simulink model "mpc_utarget"  (Simulink 6.0)
settings: Solver=ode45  SolverMode=SingleTasking  StartTime=0.0  StopTime=5  RelTol=1e-3
values from neighbouring files (symbols this model uses):
  A = sys.a    [misosim.m]    (also in mpcutarget.m)
  B = sys.b    [misosim.m]    (also in mpcutarget.m)
  C = sys.c    [misosim.m]    (also in mpcutarget.m)
  D = sys.d    [misosim.m]    (also in mpcutarget.m)
  x0 = [0 0 0 0 0]'    [misosim.m]    (also in mpcmotormodel.m = zeros(4,1); mpcoutputconstr.m = [0 0]'; mpcpreview.m = [0 0 0]'; mpcutarget.m = [0 0 0 0]')
libraries: mpclib x1
settings Model: Creator=jowen  LastModifiedBy=jowen  ExtModeTrigMode=oneshot  ExtModeArmWhenConnect=off
settings DataIOCC: LimitDataPoints=off  SignalLoggingName=sigsOut
settings OptimizationCC: BooleanDataType=off
settings DebuggingCC: CheckExecutionContextPreStartOutputMsg=on  CheckExecutionContextRuntimeOutputMsg=on  SolverPrmCheckMsg=none  IntegerOverflowMsg=none
settings HardwareCC: TargetUnknown=on
settings SFSimCC: SFSimApplyToAllLibs=on  SFSimBuildMode=Incremental

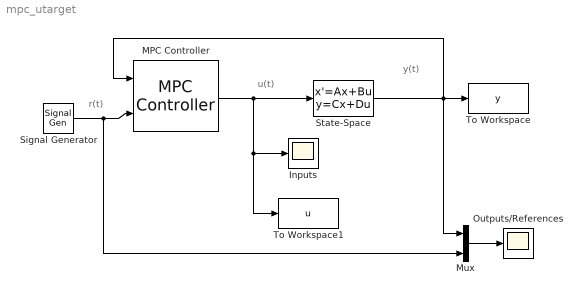
== system mpc_utarget ==
  note: u(t)
  note: y(t)
  note: r(t)
  Inputs : Scope
      settings: TimeRange=40  YMin=-4  YMax=3  DataFormat=Structure
  MPC Controller : mpclib/MPC Controller  mpcobj=mpcobj  n_mv=0  x0=[]  ref_from_ws=off  ref_signal_name=[]  ref_preview=on  md_from_ws=off  md_signal_name=[]  md_preview=on  from_project=off  md_inport=off  project_file=MPCtask.mat
  Mux : Mux  Inputs=2
  Outputs/References : Scope
      settings: TimeRange=40  YMin=-1.5  YMax=1.5  DataFormat=Structure
  Signal Generator : SignalGenerator  WaveForm=square  Frequency=.025
  State-Space : StateSpace  A=A  B=B  C=C  D=D  X0=x0
  To Workspace : ToWorkspace  VariableName=y  SampleTime=-1  SaveFormat=Array
      settings: MaxDataPoints=Inf
  To Workspace1 : ToWorkspace  VariableName=u  SampleTime=-1  SaveFormat=Array
      settings: MaxDataPoints=Inf
  wires:
  MPC Controller/1 -> State-Space/1, Inputs/1, To Workspace1/1
  State-Space/1 -> To Workspace/1, Mux/1, MPC Controller/1
  Mux/1 -> Outputs/References/1
  Signal Generator/1 -> Mux/2, MPC Controller/2
